simulink model "data_collection_surge_system"  (R2023b)
settings: Solver=VariableStepAuto  StartTime=0.0  StopTime=Tsim  RelTol=1e-3
values from neighbouring files (symbols this model uses):
  mag = 1    [surge_system.m]
  Ts = 0.1    [surge_system.m]
  x0 = (2*mx0).*rand(n,1)-mx0    [surge_system.m]
settings Model: Creator=pietrotesi  LastModifiedBy=zjhu_
settings SolverCC: AlgebraicLoopSolver=TrustRegion
settings DataIOCC: ReturnWorkspaceOutputs=off
settings DebuggingCC: UnconnectedInputMsg=warning  UnconnectedOutputMsg=warning  UnconnectedLineMsg=warning
settings ModelReferenceCC: EnableRefExpFcnMdlSchedulingChecks=on
settings RTWCC: DLArmComputeVersion=19.05

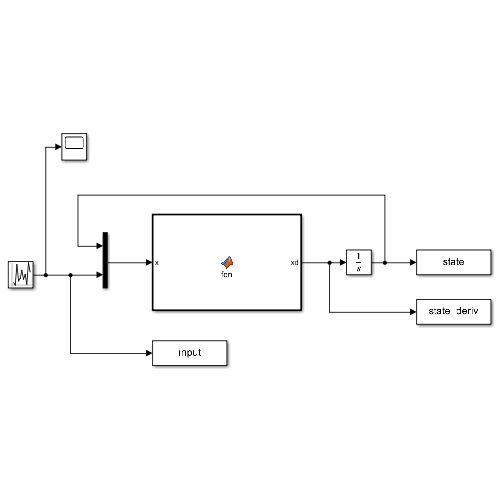
[thumbnail: Simulink's stored preview of the top-level diagram]
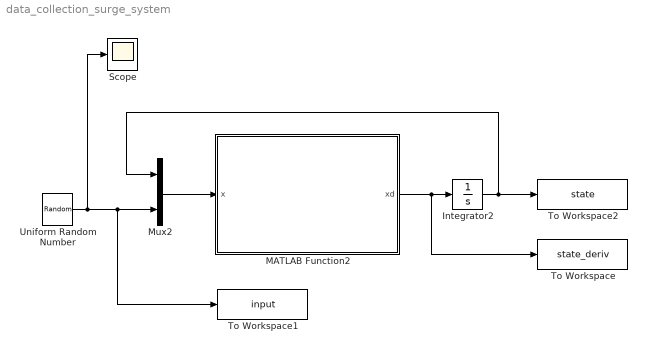
== system data_collection_surge_system ==
  Integrator2 : Integrator  InitialCondition=x0
  MATLAB Function2 : MATLAB Function  TreatAsAtomicUnit=on
  Mux2 : Mux  Inputs=2
  Scope : Scope
  To Workspace : ToWorkspace  VariableName=state_deriv  SaveFormat=Structure With Time  SampleTime=Ts
  To Workspace1 : ToWorkspace  VariableName=input  SaveFormat=Structure With Time  SampleTime=Ts
  To Workspace2 : ToWorkspace  VariableName=state  SaveFormat=Structure With Time  SampleTime=Ts
  Uniform Random Number : UniformRandomNumber  Minimum=-mag  Maximum=mag  SampleTime=Ts
  wires:
  Mux2/1 -> MATLAB Function2/1(x)
  MATLAB Function2/1(xd) -> To Workspace/1, Integrator2/1
  Uniform Random Number/1 -> Scope/1, To Workspace1/1, Mux2/2
  Integrator2/1 -> Mux2/1, To Workspace2/1

== matlab function data_collection_surge_system/MATLAB Function2 ==
  data: x input; xd output
function xd = fcn(x)

x1 = x(1);
x2 = x(2);
u = x(3);

xd = [-x2 - 1.5*x1^2 - 0.5*x1^3; u];
